simulink model "qp_torq_allocator_base"  (R2024b)
settings: Solver=VariableStepAuto  StartTime=0.0  StopTime=10.0  FixedStep=0.004  RelTol=1e-3
settings Model: Creator=lukec  LastModifiedBy=lukec
settings OptimizationCC: DefaultParameterBehavior=Inlined  EnhancedBackFolding=on  PassReuseOutputArgsAs=Individual arguments  ZeroExternalMemoryAtStartup=off  ZeroInternalMemoryAtStartup=off  OptimizeBlockOrder=speed  DifferentSizesBufferReuse=on  OptimizationCustomize=off  EfficientTunableParamExpr=on
settings DebuggingCC: ParameterTunabilityLossMsg=error
settings SFSimCC: MATLABDynamicMemAlloc=off
settings RTWCC: Description=Embedded Coder  SystemTargetFile=ert.tlc  GenCodeOnly=on  TemplateMakefile=ert_default_tmf  Toolchain=CMake  TargetLang=C++
settings CodeAppCC: ForceParamTrailComments=on  IgnoreCustomStorageClasses=off  OperatorAnnotations=on  SimulinkDataObjDesc=on  SFDataObjDesc=on  InsertBlockDesc=on
settings ERTTargetCC: TargetLangStandard=C++11 (ISO)  GenerateSampleERTMain=on  CodeInterfacePackaging=C++ class  RootIOFormat=Structure reference  ERTCustomFileTemplate=example_file_process.tlc

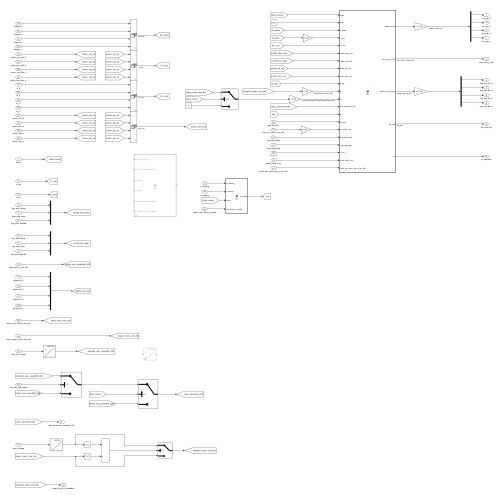
[thumbnail: Simulink's stored preview of the top-level diagram]
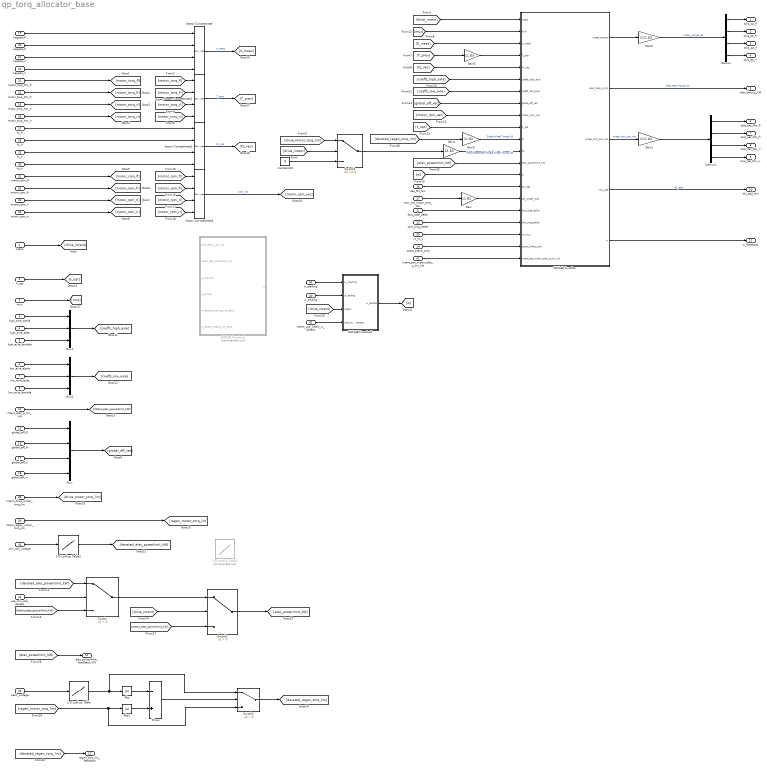
== system qp_torq_allocator_base ==
  intent : Inport
  mux : Inport  Port=2
  high_axle_alpha : Inport  Port=3
  high_axle_beta : Inport  Port=4
  high_axle_lambda : Inport  Port=5
  low_axle_alpha : Inport  Port=6
  low_axle_beta : Inport  Port=7
  low_axle_lambda : Inport  Port=8
  k_opt : Inport  Port=9
  intent_elec_p_lim_kW : Inport  Port=10
  torq_side_delta : Inport  Port=11
  torq_long_delta : Inport  Port=12
  w_starting : Inport  Port=13
  coast_brake_torq : Inport  Port=14
  global_eff_fl : Inport  Port=15
  global_eff_fr : Inport  Port=16
  global_eff_rl : Inport  Port=17
  global_eff_rr : Inport  Port=18
  kappas_fl : Inport  Port=19
  kappas_fr : Inport  Port=20
  kappas_rl : Inport  Port=21
  kappas_rr : Inport  Port=22
  motor_torq_Nm_fl : Inport  Port=23
  motor_torq_Nm_fr : Inport  Port=24
  motor_torq_Nm_rl : Inport  Port=25
  motor_torq_Nm_rr : Inport  Port=26
  fz_fl : Inport  Port=27
  fz_fr : Inport  Port=28
  fz_rl : Inport  Port=29
  fz_rr : Inport  Port=30
  motor_rpm_fl : Inport  Port=31
  motor_rpm_fr : Inport  Port=32
  motor_rpm_rl : Inport  Port=33
  motor_rpm_rr : Inport  Port=34
  vx_m_s : Inport  Port=35
  des_Mz_Nm : Inport  Port=36
  max_tot_motor_torq_Nm : Inport  Port=37
  intent_drive_motor_torq_lim : Inport  Port=38
  intent_regen_motor_torq_lim : Inport  Port=39
  w_ending : Inport  Port=40
  intent_per_motor_elec_p_lim_kW : Inport  Port=41
  intent_use_intent_w_derate : Inport  Port=42  OutDataTypeStr=boolean
  min_cell_voltage : Inport  Port=43
  use_min_cell_derate : Inport  Port=44  OutDataTypeStr=boolean
  pack_voltage : Inport  Port=45
  1-D Lookup Table : Lookup_n-D  NumberOfTableDimensions=1  BreakpointsForDimension1=[510 520]  Table=[-21 -10]  ExtrapMethod=Clip  UseLastTableValue=on  InternalRulePriority=Speed  RndMeth=Simplest
  1-D Lookup Table1 : Lookup_n-D  Commented=on  NumberOfTableDimensions=1  BreakpointsForDimension1=flip([3.5 3.3 3.1])  Table=flip([78 60 40])  ExtrapMethod=Clip  UseLastTableValue=on  InternalRulePriority=Speed  RndMeth=Simplest
  1-D Lookup Table2 : Lookup_n-D  NumberOfTableDimensions=1  BreakpointsForDimension1=flip([4.1 3.7 3.5])  Table=flip([78 60 40])  ExtrapMethod=Clip  UseLastTableValue=on  InternalRulePriority=Speed  RndMeth=Simplest
  Abs : Abs  SaturateOnIntegerOverflow=off
  Abs1 : Abs  SaturateOnIntegerOverflow=off
  Constant10 : Constant  Value=0
  Demux : Demux
  Demux1 : Demux
  Gain{,3..5} (4 alike) : Gain  Gain=11.83
  Gain1 : Gain  Gain=1/11.83
  Gain2 : Gain  Gain=1/11.83
  MATLAB Function : MATLAB Function  TreatAsAtomicUnit=on
  MATLAB Function1 : MATLAB Function  Commented=on  TreatAsAtomicUnit=on
  MATLAB Function2 : MATLAB Function  TreatAsAtomicUnit=on
  Minus : Sum  Inputs=-+
  Mux : Mux
  Mux1 : Mux  Inputs=3
  Mux2 : Mux  Inputs=3
  Switch : Switch  Criteria=u2 > Threshold  SaturateOnIntegerOverflow=off  InputSameDT=off
  Switch1 : Switch  Criteria=u2 > Threshold  SaturateOnIntegerOverflow=off  InputSameDT=off
  Switch2 : Switch  Criteria=u2 > Threshold  SaturateOnIntegerOverflow=off  InputSameDT=off
  Switch3 : Switch  SaturateOnIntegerOverflow=off  InputSameDT=off
  Vector Concatenate{,1..3} (4 alike) : Concatenate  NumInputs=4  Mode=Multidimensional array
  torq_qp_fl : Outport
  torq_qp_fr : Outport  Port=2
  torq_qp_rl : Outport  Port=3
  torq_qp_rr : Outport  Port=4
  elec_theo_p_kW : Outport  Port=5
  torq_sat_Nm_fl : Outport  Port=6
  torq_sat_Nm_fr : Outport  Port=7
  torq_sat_Nm_rl : Outport  Port=8
  torq_sat_Nm_rr : Outport  Port=9
  Mz_add_Nm : Outport  Port=10
  w_feedback : Outport  Port=11
  elec_powerlimit_feedback_kW : Outport  Port=12
  regen_torq_lim_feedback : Outport  Port=13
  wires:
  [Fz_vec] -> MATLAB Function/5(Fz_vec)
  [motor_torq_fl] -> Vector Concatenate1/1
  fz_rl/1 -> Vector Concatenate2/3
  motor_rpm_fl/1 -> [motor_rpm_fl]
  Mux/1 -> [global_eff_vec]
  [motor_torq_rl] -> Vector Concatenate1/3
  Mux2/1 -> [coeffs_low_axle]
  Vector Concatenate3/1 -> [motor_rpm_vec]  "rpm_vec"
  k_opt/1 -> [k_opt]
  Constant10/1 -> Switch3/3
  motor_rpm_rr/1 -> [motor_rpm_rr]
  Demux/4 -> torq_qp_rr/1
  des_Mz_Nm/1 -> MATLAB Function/15(Mz_des)
  fz_fl/1 -> Vector Concatenate2/1
  vx_m_s/1 -> MATLAB Function/19(vx_m_s)
  Demux/2 -> torq_qp_fr/1
  low_axle_beta/1 -> Mux2/2
  Gain5/1 -> MATLAB Function/11(lb)  "Single Wheel Torque LB"
  fz_rr/1 -> Vector Concatenate2/4
  Gain/1 -> MATLAB Function/16(tot_wheel_torq)
  motor_torq_Nm_rr/1 -> [motor_torq_rr]
  motor_rpm_rl/1 -> [motor_rpm_rl]
  [drive_intent] -> Switch3/2
  MATLAB Function/1(wheel_torque) -> Gain2/1
  MATLAB Function/2(elec_theo_p_kW) -> elec_theo_p_kW/1  "Theo. Elec. Power kW"
  fz_fr/1 -> Vector Concatenate2/2
  [motor_torq_rr] -> Vector Concatenate1/4
  motor_torq_Nm_fr/1 -> [motor_torq_fr]
  [motor_torq_fr] -> Vector Concatenate1/2
  [K_meas] -> MATLAB Function/3(K_meas)
  Switch3/1 -> Gain4/1
  Vector Concatenate/1 -> [K_meas]  "K_meas"
  high_axle_lambda/1 -> Mux1/3
  [derated_regen_torq_lim] -> Gain5/1
  global_eff_fl/1 -> Mux/1
  MATLAB Function/3(wheel_torq_sat_vec) -> Gain1/1  "wheel_torq_sat_vec"
  max_tot_motor_torq_Nm/1 -> Gain/1
  Gain4/1 -> MATLAB Function/12(ub)  "Intent Dependent Single Wheel Torque UB"
  [elec_powerlimit_kW] -> MATLAB Function/13(elec_powerlimit_kW)
  kappas_rr/1 -> Vector Concatenate/4
  intent_elec_p_lim_kW/1 -> [intent_elec_powerlimit_kW]
  high_axle_alpha/1 -> Mux1/1
  kappas_fl/1 -> Vector Concatenate/1
  low_axle_alpha/1 -> Mux2/1
  torq_side_delta/1 -> MATLAB Function/17(torq_side_delta)
  [drive_motor_torq_lim] -> Switch3/1
  Vector Concatenate2/1 -> [Fz_vec]  "Fz_vec"
  [motor_rpm_fl] -> Vector Concatenate3/1
  kappas_fr/1 -> Vector Concatenate/2
  motor_rpm_fr/1 -> [motor_rpm_fr]
  motor_torq_Nm_rl/1 -> [motor_torq_rl]
  motor_torq_Nm_fl/1 -> [motor_torq_fl]
  [motor_rpm_fr] -> Vector Concatenate3/2
  [motor_rpm_vec] -> MATLAB Function/9(motor_rpm_vec)
  low_axle_lambda/1 -> Mux2/3
  Mux1/1 -> [coeffs_high_axle]
  high_axle_beta/1 -> Mux1/2
  Gain2/1 -> Demux/1  "motor_torque_qp"
  Demux/3 -> torq_qp_rl/1
  [coeffs_low_axle] -> MATLAB Function/7(coeffs_low_axle)
  [coeffs_high_axle] -> MATLAB Function/6(coeffs_high_axle)
  [k_opt] -> MATLAB Function/10(K_opt)
  Vector Concatenate1/1 -> [T_prev]  "T_prev"
  [motor_rpm_rl] -> Vector Concatenate3/3
  kappas_rl/1 -> Vector Concatenate/3
  [global_eff_vec] -> MATLAB Function/8(global_eff_vec)
  global_eff_rl/1 -> Mux/3
  coast_brake_torq/1 -> MATLAB Function/20(coast_brake_torq)
  Demux/1 -> torq_qp_fl/1
  [drive_intent] -> MATLAB Function/1(intent)
  intent/1 -> [drive_intent]
  [motor_rpm_rr] -> Vector Concatenate3/4
  global_eff_fr/1 -> Mux/2
  Gain3/1 -> MATLAB Function/4(T_prev)
  [T_prev] -> Gain3/1
  mux/1 -> [mux]
  global_eff_rr/1 -> Mux/4
  intent_drive_motor_torq_lim/1 -> [drive_motor_torq_lim]
  intent_regen_motor_torq_lim/1 -> [regen_motor_torq_lim]
  torq_long_delta/1 -> MATLAB Function/18(torq_long_delta)
  Gain1/1 -> Demux1/1
  Demux1/1 -> torq_sat_Nm_fl/1
  Demux1/2 -> torq_sat_Nm_fr/1
  Demux1/3 -> torq_sat_Nm_rl/1
  Demux1/4 -> torq_sat_Nm_rr/1
  MATLAB Function/4(Mz_add) -> Mz_add_Nm/1  "Mz_add"
  MATLAB Function/5(w) -> w_feedback/1
  intent_per_motor_elec_p_lim_kW/1 -> MATLAB Function/21(intent_per_motor_elec_p_lim_kW)
  [mux] -> MATLAB Function/2(mux)
  w_starting/1 -> MATLAB Function2/1(w_starting)
  [drive_intent] -> MATLAB Function2/3(intent)
  w_ending/1 -> MATLAB Function2/2(w_ending)
  intent_use_intent_w_derate/1 -> MATLAB Function2/4(use_intent_w_derate)
  MATLAB Function2/1(w_derate) -> [w]
  [w] -> MATLAB Function/14("w ")
  use_min_cell_derate/1 -> Switch/2
  [derated_elec_powerlimit_kW] -> Switch/1
  [intent_elec_powerlimit_kW] -> Switch/3
  [drive_intent] -> Switch1/2
  Switch/1 -> Switch1/1
  Switch1/1 -> [elec_powerlimit_kW]
  [intent_elec_powerlimit_kW] -> Switch1/3
  [elec_powerlimit_kW] -> elec_powerlimit_feedback_kW/1
  pack_voltage/1 -> 1-D Lookup Table/1
  1-D Lookup Table/1 -> Switch2/1, Abs/1
  [regen_motor_torq_lim] -> Switch2/3, Abs1/1
  Abs/1 -> Minus/1
  Abs1/1 -> Minus/2
  Minus/1 -> Switch2/2
  Switch2/1 -> [derated_regen_torq_lim]
  min_cell_voltage/1 -> 1-D Lookup Table2/1
  1-D Lookup Table2/1 -> [derated_elec_powerlimit_kW]
  [derated_regen_torq_lim] -> regen_torq_lim_feedback/1

== matlab function qp_torq_allocator_base/MATLAB Function ==
  data: intent input; mux input; K_meas input; wheel_torque output; T_prev input; Fz_vec input; coeffs_high_axle input; coeffs_low_axle input; global_eff_vec input; motor_rpm_vec input; K_opt input; lb input; ub input; elec_theo_p_kW output; wheel_torq_sat_vec output; elec_powerlimit_kW input; w input; Mz_des input; tot_wheel_torq input; Mz_add output; torq_side_delta input; torq_long_delta input; vx_m_s input; coast_brake_torq input; w output; intent_per_motor_elec_p_lim_kW input
function [wheel_torque, elec_theo_p_kW, wheel_torq_sat_vec, Mz_add, w] = fcn(intent, mux, K_meas, T_prev, Fz_vec, coeffs_high_axle, coeffs_low_axle, global_eff_vec, motor_rpm_vec, K_opt, lb, ub, elec_powerlimit_kW, w, Mz_des, tot_wheel_torq, torq_side_delta, torq_long_delta, vx_m_s, coast_brake_torq, intent_per_motor_elec_p_lim_kW)

    % if w < 0.08
    %     w = 0.08;
    % end

    tot_wheel_torq = abs(tot_wheel_torq);

    rpm2rad_s = 0.10472;

    lb = lb .* ones(4, 1);
    ub = ub .* ones(4, 1);

    r = 0.2;
    ht = 1.2/2;

    Fz_testpoints = [-100	-150	-200	-250	-300	-350	-400	-450	-500	-550	-600	-650	-700	-750	-800	-850	-900	-950	-1000	-1050	-1100	-1150	-1200	-1250	-1300	-1350	-1400	-1450	-1500	-1550	-1600	-1650	-1700	-1750	-1800	-1850	-1900	-1950	-2000] .* -1;
    CK_testpoints = [4993.96037580768	7230.15025002608	9312.63116671493	11255.0952723015	13070.0418608112	14768.7810353328	16361.4690854774	17857.1668314117	19263.9134694458	20588.8097872709	21838.1058844771	23017.2896709141	24131.1733923846	25183.9762444061	26179.4017891894	27120.7094051015	28010.7793914951	28852.1716449660	29647.1780346286	30397.8687505021	31106.1329947657	31773.7144422382	32402.2419235013	32993.2557891554	33548.2304026337	34068.5931861850	34555.7406132517	35011.0515026319	35435.8979267288	35831.6539982093	36199.7027460456	36541.4412318642	36858.2839884342	37151.6647804853	37423.0365888119	37673.8695948128	37905.6467846387	38119.8565869283	38317.9816880605];

    CK_vec = zeros(4, 1);
    wheel_torq_peak_vec = CK_vec;

    for i = 1:4
        
        if Fz_vec(i) < min(Fz_testpoints)
            Fz_vec(i) = min(Fz_testpoints);
        elseif Fz_vec(i) > max(Fz_testpoints)
            Fz_vec(i) = max(Fz_testpoints);
        end

        CK_vec(i) = interp1(Fz_testpoints', CK_testpoints', Fz_vec(i));
        wheel_torq_peak_vec(i) = Fz_vec(i) * mux * 0.2;
    end

    peak_net_wheel_torq = sum(wheel_torq_peak_vec);
    net_fz = sum(Fz_vec);
    perc_fz = abs(Fz_vec ./ net_fz);
    wheel_torq_sat_vec = perc_fz .* peak_net_wheel_torq;

    if intent >= 0

        alpha_vec = [coeffs_low_axle(1), coeffs_low_axle(1), coeffs_high_axle(1), coeffs_high_axle(1)];
        beta_vec = [coeffs_low_axle(2), coeffs_low_axle(2), coeffs_high_axle(2), coeffs_high_axle(2)];
        lambda_vec = [coeffs_low_axle(3), coeffs_low_axle(3), coeffs_high_axle(3), coeffs_high_axle(3)];

        if abs(Mz_des) < 5 || intent > 0
            lb = 0 .* 11.83 .* ones(4, 1);
        else
            lb = coast_brake_torq .* 11.83 .* ones(4, 1);
        end

    else
        
        alpha_vec = [coeffs_high_axle(1), coeffs_high_axle(1), coeffs_low_axle(1), coeffs_low_axle(1)];
        beta_vec = [coeffs_high_axle(2), coeffs_high_axle(2), coeffs_low_axle(2), coeffs_low_axle(2)];
        lambda_vec = [coeffs_high_axle(3), coeffs_high_axle(3), coeffs_low_axle(3), coeffs_low_axle(3)];

        alpha_vec = abs(alpha_vec) .* -1;
        K_opt = abs(K_opt) * -1;
        ub = ub .* 0;

    end


    ele = zeros(4, 1);
    f = zeros(4, 1);

    for i = 1:4
        alpha = alpha_vec(i);
        beta = beta_vec(i);
        lambda = lambda_vec(i);

        CK = CK_vec(i);

        ele(i) = (beta / ((r * CK)^2)) + lambda + (w * ht^2) / (r^2);

        T_i_prev = T_prev(i);
        K_i_meas = K_meas(i);

        % term1 = -alpha * (1 / (r * CK));
        term1 = -alpha * (CK / r);

        term2_1 = (2 * (K_i_meas - K_opt)) / (r * CK);
        term2_2 = (-2 * T_i_prev) / ((r * CK)^2);
        term2 = beta * (term2_1 + term2_2);

        term3 = -2 *lambda * T_i_prev;

        f(i) = term1 + term2 + term3;
    end

    f(1) = f(1) + Mz_des * (2 * w * ht) / r;
    f(2) = f(2) - Mz_des * (2 * w * ht) / r;
    f(3) = f(3) + Mz_des * (2 * w * ht) / r;
    f(4) = f(4) - Mz_des * (2 * w * ht) / r;

    H = diag(ele) .* 2;

    % Upper off-diagonal
    H12 = (-2 * w * ht^2) / (r^2);
    H13 = (2 * w * ht^2) / (r^2);
    H14 = H12;
    H23 = H12;
    H24 = H13;
    H34 = H12;

    % Lower off-diagonal
    H21 = H12;
    H31 = H13;
    H32 = H23;
    H41 = H14;
    H42 = H24;
    H43 = H34;

    H(1, 2) = H12;
    H(1, 3) = H13;
    H(1, 4) = H14;
    H(2, 1) = H21;
    H(2, 3) = H23;
    H(2, 4) = H24;
    H(3, 1) = H31;
    H(3, 2) = H32;
    H(3, 4) = H34;
    H(4, 1) = H41;
    H(4, 2) = H42;
    H(4, 3) = H43;

    A_ine = zeros(1, 4);

    for i = 1:4
        A_ine(i) = (motor_rpm_vec(i) * rpm2rad_s / global_eff_vec(i)) / 11.83;
    end

    if intent ~= 0

        % if intent > 0
        %     lb = -3 * 11.83 .* lb;
        % end

        A_ine = [A_ine; % total power
                 diag(A_ine); % individual motor power
                 [1 1 1 1]; % total wheel torque
                 diag([1 1 1 1])]; % individual wheel saturation torque
    
        if intent < 0
            A_ine = A_ine .* -1;
        end
    
        Mz_modifier = sign(Mz_des);

        % if Mz_des == 0
        %     Mz_modifier = 0;
        % end
    

        A_ine = [A_ine;  
            [-ht/r ht/r -ht/r ht/r] .* Mz_modifier; % desired moment
            [1 -1 0 0]; % FL - FR delta 
            [-1 1 0 0]; % -FL + FR delta
            [0 0 1 -1]; % RL - RR delta 
            [0 0 -1 1]; % -RL + RR delta
            [1 0 -1 0]; % FL - RL delta 
            [-1 0 1 0]; % -FL + RL delta
            [0 1 0 -1]; % FR - RR delta 
            [0 -1 0 1]; % -FR + RR delta
            ]; 
    
        % if abs(Mz_des) <= 10
        %     torq_side_delta = 0;
        % end

        b_ine = [elec_powerlimit_kW * 1000;
                    [intent_per_motor_elec_p_lim_kW; intent_per_motor_elec_p_lim_kW; intent_per_motor_elec_p_lim_kW; intent_per_motor_elec_p_lim_kW] .* 1000;
                    tot_wheel_torq;
                    wheel_torq_sat_vec;
                    abs(Mz_des);
                    torq_side_delta * 11.83;
                    torq_side_delta * 11.83;
                    torq_side_delta * 11.83;
                    torq_side_delta * 11.83;
                    torq_long_delta * 11.83;
                    torq_long_delta * 11.83;
                    torq_long_delta * 11.83;
                    torq_long_delta * 11.83;
                    ];

        A_eq = [0 0 0 0];
        b_eq = 0;

    else

        Mz_modifier = sign(Mz_des);

        A_ine = [A_ine; % total power
                 diag(A_ine); % individual motor power
                 [1 1 1 1]; % total wheel torque
                 diag([1 1 1 1]); % individual wheel saturation torque
                 [-ht/r ht/r -ht/r ht/r] .* Mz_modifier; % desired moment
                 [1 -1 0 0]; % FL - FR delta 
                 [-1 1 0 0]; % -FL + FR delta
                 [0 0 1 -1]; % RL - RR delta 
                 [0 0 -1 1]  % -RL + RR delta
                 [1 0 -1 0]; % FL - RL delta 
                 [-1 0 1 0]; % -FL + RL delta
                 [0 1 0 -1]; % FR - RR delta 
                 [0 -1 0 1]  % -FR + RR delta
                 ]; 
    
        b_ine = [elec_powerlimit_kW * 1000;
                    [intent_per_motor_elec_p_lim_kW; intent_per_motor_elec_p_lim_kW; intent_per_motor_elec_p_lim_kW; intent_per_motor_elec_p_lim_kW] .* 1000;
                    tot_wheel_torq;
                    wheel_torq_sat_vec;
                    abs(Mz_des);
                    torq_side_delta * 11.83;
                    torq_side_delta * 11.83;
                    torq_side_delta * 11.83;
                    torq_side_delta * 11.83;
                    0 * 11.83;
                    0 * 11.83;
                    0 * 11.83;
                    0 * 11.83;
                    ];
    

        A_eq = [1 1 1 1];
        b_eq = tot_wheel_torq;

        if vx_m_s < 2 || abs(Mz_des) < 5
            ub = ub .* 0;
            lb = lb .* 0;
        end

    end
    % x0 = [0; 0; 0; 0];
    opts = optimoptions("quadprog", Algorithm="active-set");

    if intent ~= 0
        wheel_torque = quadprog(H, f, A_ine, b_ine, [], [], lb, ub, T_prev, opts);
    else
        wheel_torque = quadprog(H, f, A_ine, b_ine, A_eq, b_eq, lb, ub, T_prev, opts);
    end

    elec_theo_p_kW = (A_ine(1, :) * wheel_torque) / 1000;

    Mz_add = [-ht/r ht/r -ht/r ht/r] * wheel_torque;

    % test = lb(1);

== matlab function qp_torq_allocator_base/MATLAB Function1 ==
  data: amk_elec_p_kW_tot input; intent_elec_powerlimit_kW input; w output; w_starting input; w_ending input; w_derate_starting_kW_delta input; w_derate_ending_kW_delta input
function w = fcn(amk_elec_p_kW_tot, intent_elec_powerlimit_kW, w_starting, w_ending, w_derate_starting_kW_delta, w_derate_ending_kW_delta)

amk_elec_p_kW_tot = abs(amk_elec_p_kW_tot);
power_lb = abs(intent_elec_powerlimit_kW) - abs(w_derate_starting_kW_delta);
power_ub = abs(intent_elec_powerlimit_kW) - abs(w_derate_ending_kW_delta);

if power_lb < 0
    power_lb = 0;
end

if power_ub < 0
    power_ub = 0;
end

if power_lb == power_ub
    w = w_ending;
else
    
    if amk_elec_p_kW_tot >= power_lb

        if amk_elec_p_kW_tot > power_ub
            amk_elec_p_kW_tot = 75;
        end

        w = interp1([power_lb power_ub], [w_starting, w_ending], amk_elec_p_kW_tot);
    else
        w = w_starting;
    end

end

== matlab function qp_torq_allocator_base/MATLAB Function2 ==
  data: w_starting input; w_ending input; w_derate output; intent input; use_intent_w_derate input
function w_derate = fcn(w_starting, w_ending, intent, use_intent_w_derate)

if use_intent_w_derate

    if (intent) >= 0.9
        w_derate = interp1([0.9 1], [w_starting, w_ending], (intent));
    else
        w_derate = w_starting;
    end

else

    w_derate = w_starting;
    
end
